simulink model "problem4"  (R2019b)
settings: Solver=VariableStepAuto  StartTime=0.0  StopTime=164  RelTol=1e-3
values from neighbouring files (symbols this model uses):
  As = 4 * pi * r^2    (= 0.00125663706144)    [simulink_data.m]
  cp = 440    [simulink_data.m]
  h = 350    [simulink_data.m]
  rho = 7850    [simulink_data.m]
  Tf = 100    [simulink_data.m]
  To = 25    [simulink_data.m]
  V = 4/3 * pi * r^3    (= 4.18879020479e-06)    [simulink_data.m]
settings Model: Creator=ancar  LastModifiedBy=ancar

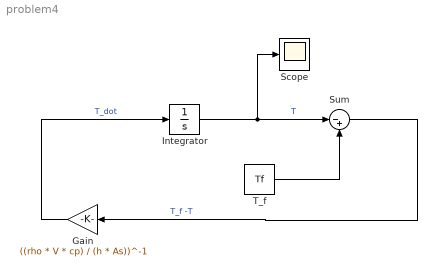
== system problem4 ==
  Gain : Gain  Gain=((rho * V * cp) / (h * As))^-1
  Integrator : Integrator  InitialCondition=To
  Scope : Scope
  Sum : Sum  Inputs=|-+
  T_f : Constant  Value=Tf
  wires:
  Gain/1 -> Integrator/1  "T_dot"
  Integrator/1 -> Scope/1, Sum/1  "T"
  T_f/1 -> Sum/2
  Sum/1 -> Gain/1  "T_f -T"
